simulink model "IEEE30_case"  (R2024b)
settings: Solver=FixedStepAuto  StartTime=0  StopTime=5  FixedStep=1e-7  RelTol=1e-3
values from neighbouring files (symbols this model uses):
  GFL_DFIG_7_C_bus = 0.08    [IEEE30_case_parameters.m]
  GFL_DFIG_7_D_mutual = 2.500000e+3    (= 2500)    [IEEE30_case_parameters.m]
  GFL_DFIG_7_f0 = 60    [IEEE30_case_parameters.m]
  GFL_DFIG_7_gPLLi = 3200    [IEEE30_case_parameters.m]
  GFL_DFIG_7_gPLLp = 650    [IEEE30_case_parameters.m]
  GFL_DFIG_7_H_WT = 0.4    [IEEE30_case_parameters.m]
  GFL_DFIG_7_Hg = 0.8    [IEEE30_case_parameters.m]
  GFL_DFIG_7_Igq_ref = 0    [IEEE30_case_parameters.m]
  GFL_DFIG_7_Ird_ref = 704.45696    [IEEE30_case_parameters.m]
  GFL_DFIG_7_KI_V = -300000    [IEEE30_case_parameters.m]
  GFL_DFIG_7_KP_V = -1000    [IEEE30_case_parameters.m]
  GFL_DFIG_7_Ksh = 1.254300e+4    (= 12543)    [IEEE30_case_parameters.m]
  GFL_DFIG_7_Lg = 0.000483    [IEEE30_case_parameters.m]
  GFL_DFIG_7_Lm_pu = 4    [IEEE30_case_parameters.m]
  GFL_DFIG_7_N = 100    [IEEE30_case_parameters.m]
  GFL_DFIG_7_p = 2    [IEEE30_case_parameters.m]
  GFL_DFIG_7_Pitch = 0    [IEEE30_case_parameters.m]
  GFL_DFIG_7_R = 44    [IEEE30_case_parameters.m]
  GFL_DFIG_7_Rg = 2.000000e-5    (= 2e-05)    [IEEE30_case_parameters.m]
  GFL_DFIG_7_rho = 1.225    [IEEE30_case_parameters.m]
  GFL_DFIG_7_rPLLi = 4500    [IEEE30_case_parameters.m]
  GFL_DFIG_7_rPLLp = 620    [IEEE30_case_parameters.m]
  GFL_DFIG_7_Rs_pu = 0.011    [IEEE30_case_parameters.m]
  GFL_DFIG_7_Sbase = 2.000000e+6    (= 2000000)    [IEEE30_case_parameters.m]
  GFL_DFIG_7_ugq_ref = 0    [IEEE30_case_parameters.m]
  GFL_DFIG_7_usd_ref = 0    [IEEE30_case_parameters.m]
  GFL_DFIG_7_Vbase = 690    [IEEE30_case_parameters.m]
  GFL_DFIG_7_Vdc_ref = 1200    [IEEE30_case_parameters.m]
  GFL_DFIG_7_wind = 12    [IEEE30_case_parameters.m]
  GFL_DFIG_7_wm_ref = 518.184209    [IEEE30_case_parameters.m]
  SG_D_13_D = 0.01056    [IEEE30_case_parameters.m]
  SG_D_13_EnableSaturation = 0    [IEEE30_case_parameters.m]
  SG_D_13_f0 = 60    [IEEE30_case_parameters.m]
  SG_D_13_H = 7.5    [IEEE30_case_parameters.m]
  SG_D_13_K_A = 20    [IEEE30_case_parameters.m]
  SG_D_13_K_E = 1.000000e+1    (= 10)    [IEEE30_case_parameters.m]
  SG_D_13_K_F = 2.363    [IEEE30_case_parameters.m]
  SG_D_13_K_s = 0.5    [IEEE30_case_parameters.m]
  SG_D_13_R_a = 0.001088    [IEEE30_case_parameters.m]
  SG_D_13_S_A = 1    [IEEE30_case_parameters.m]
  SG_D_13_S_B = 0.103    [IEEE30_case_parameters.m]
  SG_D_13_S_N = 10.659857    [IEEE30_case_parameters.m]
  SG_D_13_SpeedPara = 200    [IEEE30_case_parameters.m]
  SG_D_13_T_0 = 0.370163    [IEEE30_case_parameters.m]
  SG_D_13_T_1 = 0.3    [IEEE30_case_parameters.m]
  SG_D_13_T_2 = 0.05    [IEEE30_case_parameters.m]
  SG_D_13_T_3 = 0.02    [IEEE30_case_parameters.m]
  SG_D_13_T_4 = 0.005    [IEEE30_case_parameters.m]
  SG_D_13_T_A = 0.02    [IEEE30_case_parameters.m]
  SG_D_13_T_dd = 8.000000e+0    (= 8)    [IEEE30_case_parameters.m]
  SG_D_13_T_ddd = 0.04    [IEEE30_case_parameters.m]
  SG_D_13_T_E = 0.314    [IEEE30_case_parameters.m]
  SG_D_13_T_F = 0.35    [IEEE30_case_parameters.m]
  SG_D_13_T_qd = 0.8    [IEEE30_case_parameters.m]
  SG_D_13_T_qdd = 0.02    [IEEE30_case_parameters.m]
  SG_D_13_T_speed = 0.1    [IEEE30_case_parameters.m]
  SG_D_13_T_w = 0.5    [IEEE30_case_parameters.m]
  SG_D_13_V_ref = 1.696619    [IEEE30_case_parameters.m]
  SG_D_13_w_ref = 376.991118    [IEEE30_case_parameters.m]
  SG_D_13_x_d = 1.9    [IEEE30_case_parameters.m]
  SG_D_13_x_dd = 0.302    [IEEE30_case_parameters.m]
  SG_D_13_x_ddd = 0.204    [IEEE30_case_parameters.m]
  SG_D_13_x_l = 0.05    [IEEE30_case_parameters.m]
  SG_D_13_x_q = 1.3    [IEEE30_case_parameters.m]
  SG_D_13_x_qd = 0.5    [IEEE30_case_parameters.m]
  SG_D_13_x_qdd = 0.3    [IEEE30_case_parameters.m]
  SG_D_1_D = 0.01056    [IEEE30_case_parameters.m]
  SG_D_1_EnableSaturation = 0    [IEEE30_case_parameters.m]
  SG_D_1_f0 = 60    [IEEE30_case_parameters.m]
  SG_D_1_H = 7.5    [IEEE30_case_parameters.m]
  SG_D_1_K_A = 20    [IEEE30_case_parameters.m]
  SG_D_1_K_E = 1.000000e+1    (= 10)    [IEEE30_case_parameters.m]
  SG_D_1_K_F = 2.363    [IEEE30_case_parameters.m]
  SG_D_1_K_s = 0.5    [IEEE30_case_parameters.m]
  SG_D_1_R_a = 0.001088    [IEEE30_case_parameters.m]
  SG_D_1_S_A = 1    [IEEE30_case_parameters.m]
  SG_D_1_S_B = 0.103    [IEEE30_case_parameters.m]
  SG_D_1_S_N = 10.659857    [IEEE30_case_parameters.m]
  SG_D_1_SpeedPara = 200    [IEEE30_case_parameters.m]
  SG_D_1_T_0 = 0.259812    [IEEE30_case_parameters.m]
  SG_D_1_T_1 = 0.3    [IEEE30_case_parameters.m]
  SG_D_1_T_2 = 0.05    [IEEE30_case_parameters.m]
  SG_D_1_T_3 = 0.02    [IEEE30_case_parameters.m]
  SG_D_1_T_4 = 0.005    [IEEE30_case_parameters.m]
  SG_D_1_T_A = 0.02    [IEEE30_case_parameters.m]
  SG_D_1_T_dd = 8.000000e+0    (= 8)    [IEEE30_case_parameters.m]
  SG_D_1_T_ddd = 0.04    [IEEE30_case_parameters.m]
  SG_D_1_T_E = 0.314    [IEEE30_case_parameters.m]
  SG_D_1_T_F = 0.35    [IEEE30_case_parameters.m]
  SG_D_1_T_qd = 0.8    [IEEE30_case_parameters.m]
  SG_D_1_T_qdd = 0.02    [IEEE30_case_parameters.m]
  SG_D_1_T_speed = 0.1    [IEEE30_case_parameters.m]
  SG_D_1_T_w = 0.5    [IEEE30_case_parameters.m]
  SG_D_1_V_ref = 1.544107    [IEEE30_case_parameters.m]
  SG_D_1_w_ref = 376.991118    [IEEE30_case_parameters.m]
  SG_D_1_x_d = 1.9    [IEEE30_case_parameters.m]
  SG_D_1_x_dd = 0.302    [IEEE30_case_parameters.m]
  SG_D_1_x_ddd = 0.204    [IEEE30_case_parameters.m]
  SG_D_1_x_l = 0.05    [IEEE30_case_parameters.m]
  SG_D_1_x_q = 1.3    [IEEE30_case_parameters.m]
  SG_D_1_x_qd = 0.5    [IEEE30_case_parameters.m]
  SG_D_1_x_qdd = 0.3    [IEEE30_case_parameters.m]
  SG_D_22_D = 0.01056    [IEEE30_case_parameters.m]
  SG_D_22_EnableSaturation = 0    [IEEE30_case_parameters.m]
  SG_D_22_f0 = 60    [IEEE30_case_parameters.m]
  SG_D_22_H = 7.5    [IEEE30_case_parameters.m]
  SG_D_22_K_A = 20    [IEEE30_case_parameters.m]
  SG_D_22_K_E = 1.000000e+1    (= 10)    [IEEE30_case_parameters.m]
  SG_D_22_K_F = 2.363    [IEEE30_case_parameters.m]
  SG_D_22_K_s = 0.5    [IEEE30_case_parameters.m]
  SG_D_22_R_a = 0.001088    [IEEE30_case_parameters.m]
  SG_D_22_S_A = 1    [IEEE30_case_parameters.m]
  SG_D_22_S_B = 0.103    [IEEE30_case_parameters.m]
  SG_D_22_S_N = 10.659857    [IEEE30_case_parameters.m]
  SG_D_22_SpeedPara = 200    [IEEE30_case_parameters.m]
  SG_D_22_T_0 = 0.216121    [IEEE30_case_parameters.m]
  SG_D_22_T_1 = 0.3    [IEEE30_case_parameters.m]
  SG_D_22_T_2 = 0.05    [IEEE30_case_parameters.m]
  SG_D_22_T_3 = 0.02    [IEEE30_case_parameters.m]
  SG_D_22_T_4 = 0.005    [IEEE30_case_parameters.m]
  ... (+126 more)
(part 21 of 27)

== system IEEE30_case/SG_D_2/d_w_SG_D_2_block ==
  note: d_w_SG_D_2 in IEEE30_case
      | $\frac{2\,\pi \,T_{m,\mathrm{SG},D,2}\,f_{0}-D\,\left(w_{\mathrm{SG},D,2}-2\,\pi \,f_{0}\right)+2\,\pi \,f_{0}\,\left(\frac{\psi _{d,\mathrm{SG},D,2}\,\left(\psi _{q,\mathrm{SG},D,2}+\frac{\psi _{\mathrm{gq},\mathrm{SG},D,2}\,\left(x_{l}-x_{\mathrm{qdd}}\right)}{x_{l}-x_{\mathrm{qd}}}+\frac{\psi _{\mathrm{kq},\mathrm{SG},D,2}\,\left(x_{\mathrm{qd}}-x_{\mathrm{qdd}}\right)}{x_{l}-x_{\mathrm{qd}}}\right)}{x_{\mathrm{qdd}}}+\frac{\psi _{q,\mathrm{SG},D,2}\,\left(\frac{\psi _{\mathrm{1d},\mathrm{SG},D,2}\,\left(x_{\mathrm{dd}}-x_{\mathrm{ddd}}\right)}{x_{\mathrm{dd}}-x_{l}}-\psi _{d,\mathrm{SG},D,2}+\frac{\psi _{\mathrm{fd},\mathrm{SG},D,2}\,\left(x_{\mathrm{ddd}}-x_{l}\right)}{x_{\mathrm{dd}}-x_{l}}\right)}{x_{\mathrm{ddd}}}\right)}{2\,H}$
      | Automatically generated on 2025-11-01 18:31:31 .
  State_w_SG_D_2_071c4 : Inport
  State_T_m_SG_D_2_860e5 : Inport  Port=2
  State_psi_d_SG_D_2_34ede : Inport  Port=3
  State_psi_gq_SG_D_2_9f73e : Inport  Port=4
  State_psi_kq_SG_D_2_c590e : Inport  Port=5
  State_psi_q_SG_D_2_76d6b : Inport  Port=6
  State_psi_q_SG_D_2_b0e4a : Inport  Port=7
  State_psi_1d_SG_D_2_97ed5 : Inport  Port=8
  State_psi_d_SG_D_2_9b8cf : Inport  Port=9
  State_psi_fd_SG_D_2_66d61 : Inport  Port=10
  Add_2de3b : Sum
  Add_3480c : Sum
  Add_48811 : Sum
  Add_490e2 : Sum
  Add_ac965 : Sum
  Add_c5c05 : Sum
  Add_cbfef : Sum
  Add_e3b53 : Sum
  Constant_-1_0f227 : Constant  Value=-1
  Constant_-1_31bfd : Constant  Value=-1
  Constant_-1_403be : Constant  Value=-1
  Constant_-1_8cfa0 : Constant  Value=-1
  Constant_-1_aa771 : Constant  Value=-1
  Constant_-1_c9d01 : Constant  Value=-1
  Constant_-2.0_e1ab0 : Constant  Value=-2.0
  Constant_2.0_7b2d5 : Constant  Value=2.0
  Constant_2.0_88953 : Constant  Value=2.0
  Constant_2.0_a1518 : Constant  Value=2.0
  Constant_D_aefe5 : Constant  Value=D
  Constant_H_d5073 : Constant  Value=H
  Constant_f0_92636 : Constant  Value=f0
  Constant_f0_969d1 : Constant  Value=f0
  Constant_f0_ac18e : Constant  Value=f0
  Constant_pi_a4aaa : Constant  Value=pi
  Constant_pi_ba27e : Constant  Value=pi
  Constant_pi_e4e5a : Constant  Value=pi
  Constant_x_dd_04dea : Constant  Value=x_dd
  Constant_x_dd_1dd6c : Constant  Value=x_dd
  Constant_x_dd_c91bf : Constant  Value=x_dd
  Constant_x_ddd_2aedd : Constant  Value=x_ddd
  Constant_x_ddd_ab5ce : Constant  Value=x_ddd
  Constant_x_ddd_af871 : Constant  Value=x_ddd
  Constant_x_l_51bc5 : Constant  Value=x_l
  Constant_x_l_9b514 : Constant  Value=x_l
  Constant_x_l_9de80 : Constant  Value=x_l
  Constant_x_l_b1654 : Constant  Value=x_l
  Constant_x_l_d50ef : Constant  Value=x_l
  Constant_x_l_e71a3 : Constant  Value=x_l
  Constant_x_qd_83da6 : Constant  Value=x_qd
  Constant_x_qd_c91d9 : Constant  Value=x_qd
  Constant_x_qd_f6865 : Constant  Value=x_qd
  Constant_x_qdd_13a68 : Constant  Value=x_qdd
  Constant_x_qdd_65572 : Constant  Value=x_qdd
  Constant_x_qdd_d4bb8 : Constant  Value=x_qdd
  Divide_24348 : Product  Inputs=*/
  Divide_4956c : Product  Inputs=*/
  Divide_b34f4 : Product  Inputs=*/
  Divide_c5fd0 : Product  Inputs=*/
  Divide_df850 : Product  Inputs=*/
  Divide_edb71 : Product  Inputs=*/
  Divide_f021f : Product  Inputs=*/
  Product_08d4b : Product
  Product_17292 : Product
  Product_197e6 : Product
  Product_46ca4 : Product
  Product_50005 : Product
  Product_567dd : Product
  Product_57114 : Product
  Product_67bf0 : Product
  Product_775d5 : Product
  Product_7a3b7 : Product
  Product_9210e : Product
  Product_934a5 : Product
  Product_b04a5 : Product
  Product_b6084 : Product
  Product_b7d0d : Product
  Product_cd995 : Product
  Product_d2ecf : Product
  Product_deb05 : Product
  Product_e6081 : Product
  Product_e630b : Product
  Product_eaea2 : Product
  Product_ed81a : Product
  Subtract_0b144 : Sum  Inputs=+-
  Subtract_0e36e : Sum  Inputs=+-
  Subtract_4b2ef : Sum  Inputs=+-
  Subtract_59a92 : Sum  Inputs=+-
  Subtract_5b0ec : Sum  Inputs=+-
  Subtract_8ba6d : Sum  Inputs=+-
  Subtract_9d6d9 : Sum  Inputs=+-
  Subtract_b5e26 : Sum  Inputs=+-
  Blockout_d_w_SG_D_2_6b1c2 : Outport
  wires:
  Constant_x_qd_c91d9/1 -> Subtract_9d6d9/1
  Constant_-1_c9d01/1 -> Product_cd995/1
  Constant_-1_403be/1 -> Product_e630b/1
  Constant_x_qdd_65572/1 -> Subtract_9d6d9/2
  Subtract_b5e26/1 -> Divide_b34f4/2
  Constant_x_l_9b514/1 -> Product_cd995/2
  Constant_x_l_e71a3/1 -> Product_e630b/2
  Product_cd995/1 -> Add_ac965/1
  Product_e630b/1 -> Add_2de3b/1
  Constant_x_l_9de80/1 -> Subtract_4b2ef/2
  Constant_x_l_b1654/1 -> Product_b6084/2
  Constant_x_ddd_af871/1 -> Divide_24348/2
  Subtract_5b0ec/1 -> Product_934a5/2
  Constant_x_qd_f6865/1 -> Add_ac965/2
  Constant_x_qdd_d4bb8/1 -> Add_2de3b/2
  Constant_-1_aa771/1 -> Product_b6084/1
  State_psi_d_SG_D_2_34ede/1 -> Product_50005/2
  Constant_-1_8cfa0/1 -> Product_67bf0/1
  State_w_SG_D_2_071c4/1 -> Add_c5c05/2
  Product_b6084/1 -> Add_e3b53/1
  State_psi_1d_SG_D_2_97ed5/1 -> Product_67bf0/2
  Constant_x_dd_04dea/1 -> Subtract_59a92/1
  Divide_c5fd0/1 -> Subtract_0e36e/1
  Subtract_9d6d9/1 -> Product_567dd/2
  Constant_x_ddd_2aedd/1 -> Subtract_59a92/2
  State_psi_gq_SG_D_2_9f73e/1 -> Product_ed81a/1
  Add_ac965/1 -> Divide_edb71/2
  State_psi_d_SG_D_2_9b8cf/1 -> Add_cbfef/2
  Add_2de3b/1 -> Product_ed81a/2
  Constant_x_qd_83da6/1 -> Add_e3b53/2
  State_psi_kq_SG_D_2_c590e/1 -> Product_567dd/1
  Product_67bf0/1 -> Product_17292/1
  Subtract_59a92/1 -> Product_17292/2
  Constant_pi_a4aaa/1 -> Product_d2ecf/2
  Constant_x_dd_1dd6c/1 -> Subtract_4b2ef/1
  Constant_x_ddd_ab5ce/1 -> Subtract_5b0ec/1
  Constant_x_l_d50ef/1 -> Subtract_5b0ec/2
  Product_ed81a/1 -> Divide_c5fd0/1
  Add_e3b53/1 -> Divide_c5fd0/2
  Add_490e2/1 -> Product_197e6/2
  Product_567dd/1 -> Divide_edb71/1
  Constant_pi_e4e5a/1 -> Product_46ca4/2
  Product_17292/1 -> Divide_f021f/1
  Subtract_4b2ef/1 -> Divide_f021f/2
  State_psi_fd_SG_D_2_66d61/1 -> Product_934a5/1
  Divide_f021f/1 -> Add_cbfef/1
  Constant_x_dd_c91bf/1 -> Subtract_b5e26/1
  Constant_x_l_51bc5/1 -> Subtract_b5e26/2
  Divide_edb71/1 -> Subtract_0e36e/2
  Product_934a5/1 -> Divide_b34f4/1
  Constant_-1_0f227/1 -> Product_50005/1
  Constant_-2.0_e1ab0/1 -> Product_46ca4/1
  Subtract_0e36e/1 -> Add_490e2/1
  Subtract_8ba6d/1 -> Product_b7d0d/2
  State_psi_q_SG_D_2_76d6b/1 -> Add_490e2/2
  Constant_D_aefe5/1 -> Product_e6081/2
  Add_cbfef/1 -> Subtract_8ba6d/1
  Divide_b34f4/1 -> Subtract_8ba6d/2
  Product_46ca4/1 -> Product_775d5/1
  Constant_f0_92636/1 -> Product_775d5/2
  Constant_2.0_88953/1 -> Product_d2ecf/1
  Product_50005/1 -> Product_197e6/1
  State_psi_q_SG_D_2_b0e4a/1 -> Product_b7d0d/1
  Constant_-1_31bfd/1 -> Product_e6081/1
  Product_775d5/1 -> Add_c5c05/1
  Product_d2ecf/1 -> Product_08d4b/1
  State_T_m_SG_D_2_860e5/1 -> Product_08d4b/2
  Constant_2.0_a1518/1 -> Product_9210e/1
  Constant_pi_ba27e/1 -> Product_9210e/2
  Product_197e6/1 -> Divide_df850/1
  Constant_x_qdd_13a68/1 -> Divide_df850/2
  Product_b7d0d/1 -> Divide_24348/1
  Product_e6081/1 -> Product_eaea2/1
  Add_c5c05/1 -> Product_eaea2/2
  Product_08d4b/1 -> Product_57114/1
  Constant_f0_ac18e/1 -> Product_57114/2
  Product_9210e/1 -> Product_deb05/1
  Constant_f0_969d1/1 -> Product_deb05/2
  Divide_df850/1 -> Add_3480c/1
  Divide_24348/1 -> Add_3480c/2
  Product_eaea2/1 -> Add_48811/1
  Product_57114/1 -> Add_48811/2
  Product_deb05/1 -> Product_7a3b7/1
  Add_3480c/1 -> Product_7a3b7/2
  Add_48811/1 -> Subtract_0b144/1
  Product_7a3b7/1 -> Subtract_0b144/2
  Constant_2.0_7b2d5/1 -> Product_b04a5/1
  Constant_H_d5073/1 -> Product_b04a5/2
  Subtract_0b144/1 -> Divide_4956c/1
  Product_b04a5/1 -> Divide_4956c/2
  Divide_4956c/1 -> Blockout_d_w_SG_D_2_6b1c2/1

== system IEEE30_case/SG_D_2/i_d_SG_D_2_block ==
  note: i_d_SG_D_2 in IEEE30_case
      | $\frac{\sin\left(\theta _{\mathrm{SG},D,2}\right)\,\left(\frac{\psi _{\mathrm{1d},\mathrm{SG},D,2}\,\left(x_{\mathrm{dd}}-x_{\mathrm{ddd}}\right)}{x_{\mathrm{dd}}-x_{l}}-\psi _{d,\mathrm{SG},D,2}+\frac{\psi _{\mathrm{fd},\mathrm{SG},D,2}\,\left(x_{\mathrm{ddd}}-x_{l}\right)}{x_{\mathrm{dd}}-x_{l}}\right)}{x_{\mathrm{ddd}}}-\frac{\cos\left(\theta _{\mathrm{SG},D,2}\right)\,\left(\psi _{q,\mathrm{SG},D,2}+\frac{\psi _{\mathrm{gq},\mathrm{SG},D,2}\,\left(x_{l}-x_{\mathrm{qdd}}\right)}{x_{l}-x_{\mathrm{qd}}}+\frac{\psi _{\mathrm{kq},\mathrm{SG},D,2}\,\left(x_{\mathrm{qd}}-x_{\mathrm{qdd}}\right)}{x_{l}-x_{\mathrm{qd}}}\right)}{x_{\mathrm{qdd}}}$
      | Automatically generated on 2025-11-01 18:31:53 .
  State_psi_gq_SG_D_2_ef87c : Inport
  State_psi_kq_SG_D_2_da414 : Inport  Port=2
  State_psi_q_SG_D_2_14a65 : Inport  Port=3
  State_theta_SG_D_2_b0b05 : Inport  Port=4
  State_psi_1d_SG_D_2_baa39 : Inport  Port=5
  State_psi_d_SG_D_2_956af : Inport  Port=6
  State_psi_fd_SG_D_2_52aed : Inport  Port=7
  State_theta_SG_D_2_57fa8 : Inport  Port=8
  Add_190e7 : Sum
  Add_2cec0 : Sum
  Add_5ba1c : Sum
  Add_e5908 : Sum
  Add_f3d0a : Sum
  Constant_-1_2e41f : Constant  Value=-1
  Constant_-1_404a3 : Constant  Value=-1
  Constant_-1_80a87 : Constant  Value=-1
  Constant_-1_f25b1 : Constant  Value=-1
  Constant_-1_f5693 : Constant  Value=-1
  Constant_x_dd_2d4e9 : Constant  Value=x_dd
  Constant_x_dd_42557 : Constant  Value=x_dd
  Constant_x_dd_b8c41 : Constant  Value=x_dd
  Constant_x_ddd_2c46a : Constant  Value=x_ddd
  Constant_x_ddd_8aad1 : Constant  Value=x_ddd
  Constant_x_ddd_95243 : Constant  Value=x_ddd
  Constant_x_l_08223 : Constant  Value=x_l
  Constant_x_l_355f8 : Constant  Value=x_l
  Constant_x_l_559b2 : Constant  Value=x_l
  Constant_x_l_b22e8 : Constant  Value=x_l
  Constant_x_l_d52ee : Constant  Value=x_l
  Constant_x_l_e61e2 : Constant  Value=x_l
  Constant_x_qd_3c262 : Constant  Value=x_qd
  Constant_x_qd_5b82d : Constant  Value=x_qd
  Constant_x_qd_da69c : Constant  Value=x_qd
  Constant_x_qdd_1f1d5 : Constant  Value=x_qdd
  Constant_x_qdd_3610f : Constant  Value=x_qdd
  Constant_x_qdd_cad96 : Constant  Value=x_qdd
  Divide_32941 : Product  Inputs=*/
  Divide_3dcdd : Product  Inputs=*/
  Divide_9da8b : Product  Inputs=*/
  Divide_aeac0 : Product  Inputs=*/
  Divide_c0da5 : Product  Inputs=*/
  Divide_e74a2 : Product  Inputs=*/
  MathFunc_cos_8df34 : Trigonometry  Operator=cos
  MathFunc_sin_f790c : Trigonometry
  Product_11a30 : Product
  Product_11e29 : Product
  Product_2653c : Product
  Product_2b1e0 : Product
  Product_3265d : Product
  Product_3d1f3 : Product
  Product_4bdee : Product
  Product_60792 : Product
  Product_af2fe : Product
  Product_ba15b : Product
  Product_d1e53 : Product
  Subtract_38201 : Sum  Inputs=+-
  Subtract_4005b : Sum  Inputs=+-
  Subtract_7917b : Sum  Inputs=+-
  Subtract_90c1d : Sum  Inputs=+-
  Subtract_9241a : Sum  Inputs=+-
  Subtract_92dc1 : Sum  Inputs=+-
  Subtract_b4de5 : Sum  Inputs=+-
  Subtract_e026e : Sum  Inputs=+-
  Blockout_i_d_SG_D_2_ae2df : Outport
  wires:
  Constant_x_ddd_2c46a/1 -> Subtract_b4de5/1
  Constant_x_qd_da69c/1 -> Subtract_38201/1
  Constant_-1_80a87/1 -> Product_af2fe/1
  Constant_-1_f25b1/1 -> Product_3d1f3/1
  Subtract_9241a/1 -> Blockout_i_d_SG_D_2_ae2df/1
  Constant_x_qdd_cad96/1 -> Subtract_38201/2
  Constant_x_l_b22e8/1 -> Product_af2fe/2
  Constant_x_l_559b2/1 -> Product_3d1f3/2
  Product_af2fe/1 -> Add_f3d0a/1
  Product_3d1f3/1 -> Add_2cec0/1
  Constant_x_l_355f8/1 -> Product_2b1e0/2
  Constant_x_qd_5b82d/1 -> Add_f3d0a/2
  Constant_x_qdd_3610f/1 -> Add_2cec0/2
  Constant_x_qdd_1f1d5/1 -> Divide_c0da5/2
  MathFunc_cos_8df34/1 -> Product_3265d/2
  Constant_-1_404a3/1 -> Product_2b1e0/1
  State_psi_gq_SG_D_2_ef87c/1 -> Product_4bdee/1
  Subtract_b4de5/1 -> Product_11e29/2
  Product_ba15b/1 -> Product_2653c/1
  Add_f3d0a/1 -> Divide_9da8b/2
  Add_2cec0/1 -> Product_4bdee/2
  Product_11e29/1 -> Divide_3dcdd/1
  Product_2b1e0/1 -> Add_5ba1c/1
  Constant_x_qd_3c262/1 -> Add_5ba1c/2
  State_theta_SG_D_2_57fa8/1 -> MathFunc_sin_f790c/1
  State_psi_kq_SG_D_2_da414/1 -> Product_60792/1
  Add_190e7/1 -> Subtract_92dc1/1
  Subtract_38201/1 -> Product_60792/2
  Product_4bdee/1 -> Divide_e74a2/1
  Constant_-1_f5693/1 -> Product_ba15b/1
  State_psi_1d_SG_D_2_baa39/1 -> Product_ba15b/2
  State_psi_fd_SG_D_2_52aed/1 -> Product_11e29/1
  Constant_x_dd_b8c41/1 -> Subtract_e026e/1
  Product_2653c/1 -> Divide_aeac0/1
  Constant_x_ddd_95243/1 -> Subtract_e026e/2
  Divide_3dcdd/1 -> Subtract_92dc1/2
  Add_5ba1c/1 -> Divide_e74a2/2
  Product_11a30/1 -> Divide_32941/1
  Product_60792/1 -> Divide_9da8b/1
  Constant_-1_2e41f/1 -> Product_d1e53/1
  Subtract_4005b/1 -> Divide_3dcdd/2
  Subtract_e026e/1 -> Product_2653c/2
  Constant_x_dd_2d4e9/1 -> Subtract_7917b/1
  Subtract_92dc1/1 -> Product_11a30/1
  Constant_x_l_d52ee/1 -> Subtract_7917b/2
  Constant_x_l_08223/1 -> Subtract_b4de5/2
  Divide_e74a2/1 -> Subtract_90c1d/1
  Divide_32941/1 -> Subtract_9241a/2
  Divide_9da8b/1 -> Subtract_90c1d/2
  Subtract_7917b/1 -> Divide_aeac0/2
  Constant_x_dd_42557/1 -> Subtract_4005b/1
  Divide_c0da5/1 -> Subtract_9241a/1
  Constant_x_l_e61e2/1 -> Subtract_4005b/2
  Subtract_90c1d/1 -> Add_e5908/1
  State_psi_q_SG_D_2_14a65/1 -> Add_e5908/2
  Constant_x_ddd_8aad1/1 -> Divide_32941/2
  MathFunc_sin_f790c/1 -> Product_11a30/2
  Divide_aeac0/1 -> Add_190e7/1
  State_psi_d_SG_D_2_956af/1 -> Add_190e7/2
  Add_e5908/1 -> Product_d1e53/2
  State_theta_SG_D_2_b0b05/1 -> MathFunc_cos_8df34/1
  Product_d1e53/1 -> Product_3265d/1
  Product_3265d/1 -> Divide_c0da5/1

== system IEEE30_case/SG_D_2/i_q_SG_D_2_block ==
  note: i_q_SG_D_2 in IEEE30_case
      | $-\frac{\sin\left(\theta _{\mathrm{SG},D,2}\right)\,\left(\psi _{q,\mathrm{SG},D,2}+\frac{\psi _{\mathrm{gq},\mathrm{SG},D,2}\,\left(x_{l}-x_{\mathrm{qdd}}\right)}{x_{l}-x_{\mathrm{qd}}}+\frac{\psi _{\mathrm{kq},\mathrm{SG},D,2}\,\left(x_{\mathrm{qd}}-x_{\mathrm{qdd}}\right)}{x_{l}-x_{\mathrm{qd}}}\right)}{x_{\mathrm{qdd}}}-\frac{\cos\left(\theta _{\mathrm{SG},D,2}\right)\,\left(\frac{\psi _{\mathrm{1d},\mathrm{SG},D,2}\,\left(x_{\mathrm{dd}}-x_{\mathrm{ddd}}\right)}{x_{\mathrm{dd}}-x_{l}}-\psi _{d,\mathrm{SG},D,2}+\frac{\psi _{\mathrm{fd},\mathrm{SG},D,2}\,\left(x_{\mathrm{ddd}}-x_{l}\right)}{x_{\mathrm{dd}}-x_{l}}\right)}{x_{\mathrm{ddd}}}$
      | Automatically generated on 2025-11-01 18:31:57 .
  State_psi_gq_SG_D_2_0f140 : Inport
  State_psi_kq_SG_D_2_8caff : Inport  Port=2
  State_psi_q_SG_D_2_c9d02 : Inport  Port=3
  State_theta_SG_D_2_99776 : Inport  Port=4
  State_psi_1d_SG_D_2_3670e : Inport  Port=5
  State_psi_d_SG_D_2_82684 : Inport  Port=6
  State_psi_fd_SG_D_2_4cfda : Inport  Port=7
  State_theta_SG_D_2_e3ac6 : Inport  Port=8
  Add_18b6d : Sum
  Add_1d44b : Sum
  Add_3a2b5 : Sum
  Add_9698d : Sum
  Add_9d5bd : Sum
  Add_e2752 : Sum
  Constant_-1_{46827,56218,94343,94462} (4 alike) : Constant  Value=-1
  Constant_-1_50b0c : Constant  Value=-1
  Constant_x_dd_09e07 : Constant  Value=x_dd
  Constant_x_dd_77471 : Constant  Value=x_dd
  Constant_x_dd_79e24 : Constant  Value=x_dd
  Constant_x_ddd_2d654 : Constant  Value=x_ddd
  Constant_x_ddd_4337c : Constant  Value=x_ddd
  Constant_x_ddd_5f735 : Constant  Value=x_ddd
  Constant_x_l_433ef : Constant  Value=x_l
  Constant_x_l_4ca2f : Constant  Value=x_l
  Constant_x_l_5195e : Constant  Value=x_l
  Constant_x_l_a3f6e : Constant  Value=x_l
  Constant_x_l_ab249 : Constant  Value=x_l
  Constant_x_l_b7b4e : Constant  Value=x_l
  Constant_x_qd_4d715 : Constant  Value=x_qd
  Constant_x_qd_58a0f : Constant  Value=x_qd
  Constant_x_qd_6d9e4 : Constant  Value=x_qd
  Constant_x_qdd_3f9be : Constant  Value=x_qdd
  Constant_x_qdd_ae7a5 : Constant  Value=x_qdd
  Constant_x_qdd_ebd74 : Constant  Value=x_qdd
  Divide_05f23 : Product  Inputs=*/
  Divide_2a0fd : Product  Inputs=*/
  Divide_4fdbe : Product  Inputs=*/
  Divide_6d0b3 : Product  Inputs=*/
  Divide_b374c : Product  Inputs=*/
  Divide_f150f : Product  Inputs=*/
  MathFunc_cos_a52ff : Trigonometry  Operator=cos
  MathFunc_sin_0fb9d : Trigonometry
  Product_02529 : Product
  Product_03870 : Product
  Product_2e37c : Product
  Product_4d747 : Product
  Product_4d981 : Product
  Product_59f12 : Product
  Product_a5dfa : Product
  Product_ad008 : Product
  Product_b383d : Product
  Product_f4942 : Product
  Product_f5289 : Product
  Subtract_01e2a : Sum  Inputs=+-
  Subtract_1994f : Sum  Inputs=+-
  Subtract_608a5 : Sum  Inputs=+-
  Subtract_78221 : Sum  Inputs=+-
  Subtract_a0408 : Sum  Inputs=+-
  Subtract_abee3 : Sum  Inputs=+-
  Subtract_e9404 : Sum  Inputs=+-
  Blockout_i_q_SG_D_2_865bf : Outport
  wires:
  MathFunc_sin_0fb9d/1 -> Product_f4942/2
  Product_b383d/1 -> Product_f4942/1
  Constant_-1_56218/1 -> Product_ad008/1
  Constant_-1_94462/1 -> Product_2e37c/1
  Constant_x_l_a3f6e/1 -> Product_ad008/2
  Product_ad008/1 -> Add_9d5bd/1
  Subtract_78221/1 -> Product_03870/2
  Constant_x_qdd_ebd74/1 -> Subtract_1994f/2
  Constant_x_qdd_3f9be/1 -> Add_9d5bd/2
  Add_3a2b5/1 -> Product_b383d/2
  Constant_x_l_4ca2f/1 -> Product_2e37c/2
  Constant_x_qd_6d9e4/1 -> Subtract_1994f/1
  Constant_-1_46827/1 -> Product_59f12/1
  Constant_x_l_433ef/1 -> Product_59f12/2
  State_psi_1d_SG_D_2_3670e/1 -> Product_a5dfa/2
  State_psi_gq_SG_D_2_0f140/1 -> Product_02529/1
  Add_9d5bd/1 -> Product_02529/2
  Product_2e37c/1 -> Add_1d44b/1
  Divide_05f23/1 -> Add_18b6d/1
  Constant_x_qd_58a0f/1 -> Add_1d44b/2
  State_psi_kq_SG_D_2_8caff/1 -> Product_f5289/1
  Add_9698d/1 -> Subtract_abee3/1
  Constant_x_ddd_4337c/1 -> Subtract_78221/2
  Subtract_1994f/1 -> Product_f5289/2
  Product_59f12/1 -> Add_e2752/1
  Constant_x_qd_4d715/1 -> Add_e2752/2
  Constant_-1_94343/1 -> Product_a5dfa/1
  Constant_x_l_b7b4e/1 -> Subtract_e9404/2
  Constant_x_dd_79e24/1 -> Subtract_78221/1
  Product_02529/1 -> Divide_6d0b3/1
  Divide_4fdbe/1 -> Subtract_abee3/2
  Add_1d44b/1 -> Divide_6d0b3/2
  Product_4d981/1 -> Divide_b374c/1
  Product_f5289/1 -> Divide_f150f/1
  Constant_-1_50b0c/1 -> Product_b383d/1
  Product_a5dfa/1 -> Product_03870/1
  Add_e2752/1 -> Divide_f150f/2
  Constant_x_dd_77471/1 -> Subtract_608a5/1
  Subtract_abee3/1 -> Product_4d981/1
  Subtract_01e2a/1 -> Product_4d747/2
  Constant_x_l_5195e/1 -> Subtract_608a5/2
  Constant_x_ddd_5f735/1 -> Subtract_01e2a/1
  Constant_x_l_ab249/1 -> Subtract_01e2a/2
  Divide_6d0b3/1 -> Subtract_a0408/1
  Divide_b374c/1 -> Add_18b6d/2
  Product_4d747/1 -> Divide_4fdbe/1
  Divide_f150f/1 -> Subtract_a0408/2
  Subtract_e9404/1 -> Divide_4fdbe/2
  Product_03870/1 -> Divide_2a0fd/1
  Subtract_608a5/1 -> Divide_2a0fd/2
  Constant_x_qdd_ae7a5/1 -> Divide_05f23/2
  State_psi_fd_SG_D_2_4cfda/1 -> Product_4d747/1
  Constant_x_dd_09e07/1 -> Subtract_e9404/1
  Subtract_a0408/1 -> Add_3a2b5/1
  State_psi_q_SG_D_2_c9d02/1 -> Add_3a2b5/2
  Constant_x_ddd_2d654/1 -> Divide_b374c/2
  Divide_2a0fd/1 -> Add_9698d/1
  State_psi_d_SG_D_2_82684/1 -> Add_9698d/2
  State_theta_SG_D_2_99776/1 -> MathFunc_sin_0fb9d/1
  State_theta_SG_D_2_e3ac6/1 -> MathFunc_cos_a52ff/1
  MathFunc_cos_a52ff/1 -> Product_4d981/2
  Product_f4942/1 -> Divide_05f23/1
  Add_18b6d/1 -> Blockout_i_q_SG_D_2_865bf/1

== system IEEE30_case/SG_D_2/theta_SG_D_2_out_block ==
  note: theta_SG_D_2_out in IEEE30_case
      | $\theta _{\mathrm{SG},D,2}$
      | Automatically generated on 2025-11-01 18:32:02 .
  State_theta_SG_D_2_1ecf4 : Inport
  Blockout_theta_SG_D_2_out_e958d : Outport
  wires:
  State_theta_SG_D_2_1ecf4/1 -> Blockout_theta_SG_D_2_out_e958d/1

== system IEEE30_case/SG_D_2/w_SG_D_2_out_block ==
  note: w_SG_D_2_out in IEEE30_case
      | $w_{\mathrm{SG},D,2}$
      | Automatically generated on 2025-11-01 18:32:02 .
  State_w_SG_D_2_6b0c6 : Inport
  Blockout_w_SG_D_2_out_ca3f3 : Outport
  wires:
  State_w_SG_D_2_6b0c6/1 -> Blockout_w_SG_D_2_out_ca3f3/1

== system IEEE30_case/SG_D_22/T_e_SG_D_22_block ==
  note: T_e_SG_D_22 in IEEE30_case
      | $-\frac{\psi _{d,\mathrm{SG},D,22}\,\left(\psi _{q,\mathrm{SG},D,22}+\frac{\psi _{\mathrm{gq},\mathrm{SG},D,22}\,\left(x_{l}-x_{\mathrm{qdd}}\right)}{x_{l}-x_{\mathrm{qd}}}+\frac{\psi _{\mathrm{kq},\mathrm{SG},D,22}\,\left(x_{\mathrm{qd}}-x_{\mathrm{qdd}}\right)}{x_{l}-x_{\mathrm{qd}}}\right)}{x_{\mathrm{qdd}}}-\frac{\psi _{q,\mathrm{SG},D,22}\,\left(\frac{\psi _{\mathrm{1d},\mathrm{SG},D,22}\,\left(x_{\mathrm{dd}}-x_{\mathrm{ddd}}\right)}{x_{\mathrm{dd}}-x_{l}}-\psi _{d,\mathrm{SG},D,22}+\frac{\psi _{\mathrm{fd},\mathrm{SG},D,22}\,\left(x_{\mathrm{ddd}}-x_{l}\right)}{x_{\mathrm{dd}}-x_{l}}\right)}{x_{\mathrm{ddd}}}$
      | Automatically generated on 2025-11-01 18:36:46 .
  State_psi_d_SG_D_22_b0899 : Inport
  State_psi_gq_SG_D_22_ecb3d : Inport  Port=2
  State_psi_kq_SG_D_22_80cd8 : Inport  Port=3
  State_psi_q_SG_D_22_f98a6 : Inport  Port=4
  State_psi_q_SG_D_22_21d92 : Inport  Port=5
  State_psi_1d_SG_D_22_9ed94 : Inport  Port=6
  State_psi_d_SG_D_22_2f3ed : Inport  Port=7
  State_psi_fd_SG_D_22_d61c9 : Inport  Port=8
  Add_47e65 : Sum
  Add_5302b : Sum
  Add_7b312 : Sum
  Add_ac404 : Sum
  Add_e5157 : Sum
  Add_e840c : Sum
  Constant_-1_3e949 : Constant  Value=-1
  Constant_-1_7eaa8 : Constant  Value=-1
  Constant_-1_8f5ee : Constant  Value=-1
  Constant_-1_97a88 : Constant  Value=-1
  Constant_-1_c3af5 : Constant  Value=-1
  Constant_x_dd_87738 : Constant  Value=x_dd
  Constant_x_dd_987cc : Constant  Value=x_dd
  Constant_x_dd_e91a2 : Constant  Value=x_dd
  Constant_x_ddd_0b8f0 : Constant  Value=x_ddd
  Constant_x_ddd_2c262 : Constant  Value=x_ddd
  Constant_x_ddd_30aa0 : Constant  Value=x_ddd
  Constant_x_l_0422d : Constant  Value=x_l
  Constant_x_l_55ed8 : Constant  Value=x_l
  Constant_x_l_7dac2 : Constant  Value=x_l
  Constant_x_l_86146 : Constant  Value=x_l
  Constant_x_l_8c951 : Constant  Value=x_l
  Constant_x_l_b9baf : Constant  Value=x_l
  Constant_x_qd_97f19 : Constant  Value=x_qd
  Constant_x_qd_a1fc9 : Constant  Value=x_qd
  Constant_x_qd_a3274 : Constant  Value=x_qd
  Constant_x_qdd_71a58 : Constant  Value=x_qdd
  Constant_x_qdd_7a6a2 : Constant  Value=x_qdd
  Constant_x_qdd_bebc5 : Constant  Value=x_qdd
  Divide_02e83 : Product  Inputs=*/
  Divide_181c4 : Product  Inputs=*/
  Divide_adde5 : Product  Inputs=*/
  Divide_af1d6 : Product  Inputs=*/
  Divide_e0e20 : Product  Inputs=*/
  Divide_e1700 : Product  Inputs=*/
  Product_0f751 : Product
  Product_1571a : Product
  Product_35cfc : Product
  Product_48560 : Product
  Product_496b4 : Product
  Product_6bc40 : Product
  Product_88d29 : Product
  Product_9e9d2 : Product
  Product_9ecd4 : Product
  Product_d4864 : Product
  Product_d644d : Product
  Subtract_22c35 : Sum  Inputs=+-
  Subtract_2c2cb : Sum  Inputs=+-
  Subtract_53c24 : Sum  Inputs=+-
  Subtract_67b86 : Sum  Inputs=+-
  Subtract_7043c : Sum  Inputs=+-
  Subtract_a7308 : Sum  Inputs=+-
  Subtract_ab449 : Sum  Inputs=+-
  Blockout_T_e_SG_D_22_9d77c : Outport
  wires:
  State_psi_1d_SG_D_22_9ed94/1 -> Product_d644d/2
  Constant_-1_97a88/1 -> Product_496b4/1
  Subtract_a7308/1 -> Product_9e9d2/2
  Constant_x_ddd_0b8f0/1 -> Subtract_53c24/2
  Constant_x_l_55ed8/1 -> Product_496b4/2
  Constant_x_qd_a1fc9/1 -> Subtract_a7308/1
  Constant_x_l_0422d/1 -> Subtract_22c35/2
  Product_496b4/1 -> Add_47e65/1
  Constant_x_qdd_7a6a2/1 -> Subtract_a7308/2
  Add_ac404/1 -> Subtract_ab449/1
  Constant_x_l_8c951/1 -> Subtract_67b86/2
  Constant_x_qdd_71a58/1 -> Add_47e65/2
  Product_0f751/1 -> Add_7b312/1
  Constant_-1_3e949/1 -> Product_0f751/1
  Constant_x_l_b9baf/1 -> Product_0f751/2
  Product_6bc40/1 -> Add_e840c/1
  Constant_-1_8f5ee/1 -> Product_6bc40/1
  Constant_x_l_86146/1 -> Product_6bc40/2
  Product_d644d/1 -> Product_88d29/1
  Constant_-1_c3af5/1 -> Product_d644d/1
  Subtract_53c24/1 -> Product_88d29/2
  Constant_x_dd_87738/1 -> Subtract_53c24/1
  State_psi_gq_SG_D_22_ecb3d/1 -> Product_9ecd4/1
  Divide_181c4/1 -> Add_e5157/2
  Add_47e65/1 -> Product_9ecd4/2
  Constant_x_qd_97f19/1 -> Add_7b312/2
  Product_9e9d2/1 -> Divide_adde5/1
  Product_9ecd4/1 -> Divide_e0e20/1
  State_psi_kq_SG_D_22_80cd8/1 -> Product_9e9d2/1
  Divide_02e83/1 -> Add_ac404/1
  Constant_x_qd_a3274/1 -> Add_e840c/2
  Subtract_67b86/1 -> Divide_02e83/2
  Constant_x_dd_987cc/1 -> Subtract_67b86/1
  Constant_x_qdd_bebc5/1 -> Divide_af1d6/2
  Subtract_22c35/1 -> Product_1571a/2
  Constant_x_ddd_30aa0/1 -> Subtract_22c35/1
  Add_7b312/1 -> Divide_e0e20/2
  Add_e840c/1 -> Divide_adde5/2
  Add_e5157/1 -> Blockout_T_e_SG_D_22_9d77c/1
  Product_88d29/1 -> Divide_02e83/1
  Product_1571a/1 -> Divide_e1700/1
  State_psi_fd_SG_D_22_d61c9/1 -> Product_1571a/1
  Subtract_7043c/1 -> Divide_e1700/2
  Constant_x_dd_e91a2/1 -> Subtract_7043c/1
  Divide_e0e20/1 -> Subtract_2c2cb/1
  Constant_x_l_7dac2/1 -> Subtract_7043c/2
  Divide_adde5/1 -> Subtract_2c2cb/2
  Product_35cfc/1 -> Divide_181c4/1
  State_psi_q_SG_D_22_21d92/1 -> Product_35cfc/1
  State_psi_d_SG_D_22_2f3ed/1 -> Add_ac404/2
  Constant_-1_7eaa8/1 -> Product_48560/1
  Product_48560/1 -> Product_d4864/1
  State_psi_d_SG_D_22_b0899/1 -> Product_48560/2
  State_psi_q_SG_D_22_f98a6/1 -> Add_5302b/2
  Subtract_2c2cb/1 -> Add_5302b/1
  Divide_af1d6/1 -> Add_e5157/1
  Product_d4864/1 -> Divide_af1d6/1
  Divide_e1700/1 -> Subtract_ab449/2
  Add_5302b/1 -> Product_d4864/2
  Subtract_ab449/1 -> Product_35cfc/2
  Constant_x_ddd_2c262/1 -> Divide_181c4/2

== system IEEE30_case/SG_D_22/d_E_fd_SG_D_22_block ==
  note: d_E_fd_SG_D_22 in IEEE30_case
      | $\frac{V_{f,\mathrm{SG},D,22}-E_{\mathrm{fd},\mathrm{SG},D,22}\,K_{E}}{T_{E}}$
      | Automatically generated on 2025-11-01 18:36:29 .
  State_E_fd_SG_D_22_b7fa0 : Inport
  State_V_f_SG_D_22_c66fa : Inport  Port=2
  Add_0014f : Sum
  Constant_-1_7ae50 : Constant  Value=-1
  Constant_K_E_36d69 : Constant  Value=K_E
  Constant_T_E_84d6f : Constant  Value=T_E
  Divide_9c9c4 : Product  Inputs=*/
  Product_2266f : Product
  Product_2289b : Product
  Blockout_d_E_fd_SG_D_22_040cd : Outport
  wires:
  State_V_f_SG_D_22_c66fa/1 -> Add_0014f/2
  State_E_fd_SG_D_22_b7fa0/1 -> Product_2266f/2
  Constant_-1_7ae50/1 -> Product_2266f/1
  Constant_T_E_84d6f/1 -> Divide_9c9c4/2
  Product_2266f/1 -> Product_2289b/1
  Constant_K_E_36d69/1 -> Product_2289b/2
  Add_0014f/1 -> Divide_9c9c4/1
  Product_2289b/1 -> Add_0014f/1
  Divide_9c9c4/1 -> Blockout_d_E_fd_SG_D_22_040cd/1

== system IEEE30_case/SG_D_22/d_Px_1_SG_D_22_block ==
  note: d_Px_1_SG_D_22 in IEEE30_case
      | $\frac{w_{\mathrm{SG},D,22}-2\,\pi \,f_{0}}{T_{w}}-\frac{\mathrm{Px}_{1,\mathrm{SG},D,22}}{T_{w}}$
      | Automatically generated on 2025-11-01 18:36:30 .
  State_Px_1_SG_D_22_97642 : Inport
  State_w_SG_D_22_b06b5 : Inport  Port=2
  Add_1f38f : Sum
  Add_4bcee : Sum
  Constant_-1_a0bff : Constant  Value=-1
  Constant_-2.0_5d154 : Constant  Value=-2.0
  Constant_T_w_605e1 : Constant  Value=T_w
  Constant_T_w_c6433 : Constant  Value=T_w
  Constant_f0_ff22d : Constant  Value=f0
  Constant_pi_9163d : Constant  Value=pi
  Divide_3e1c8 : Product  Inputs=*/
  Divide_8b428 : Product  Inputs=*/
  Product_1f09a : Product
  Product_70952 : Product
  Product_88b24 : Product
  Blockout_d_Px_1_SG_D_22_5a954 : Outport
  wires:
  Constant_-2.0_5d154/1 -> Product_1f09a/1
  Product_1f09a/1 -> Product_70952/1
  Constant_pi_9163d/1 -> Product_1f09a/2
  Constant_f0_ff22d/1 -> Product_70952/2
  Constant_-1_a0bff/1 -> Product_88b24/1
  Product_70952/1 -> Add_4bcee/1
  State_Px_1_SG_D_22_97642/1 -> Product_88b24/2
  State_w_SG_D_22_b06b5/1 -> Add_4bcee/2
  Product_88b24/1 -> Divide_3e1c8/1
  Constant_T_w_c6433/1 -> Divide_3e1c8/2
  Add_4bcee/1 -> Divide_8b428/1
  Constant_T_w_605e1/1 -> Divide_8b428/2
  Divide_3e1c8/1 -> Add_1f38f/1
  Divide_8b428/1 -> Add_1f38f/2
  Add_1f38f/1 -> Blockout_d_Px_1_SG_D_22_5a954/1

== system IEEE30_case/SG_D_22/d_Px_2_SG_D_22_block ==
  note: d_Px_2_SG_D_22 in IEEE30_case
      | $\frac{\mathrm{Px}_{1,\mathrm{SG},D,22}-T_{2}\,\left(\frac{\mathrm{Px}_{1,\mathrm{SG},D,22}}{T_{w}}-\frac{w_{\mathrm{SG},D,22}-2\,\pi \,f_{0}}{T_{w}}\right)}{T_{1}}-\frac{\mathrm{Px}_{2,\mathrm{SG},D,22}}{T_{1}}$
      | Automatically generated on 2025-11-01 18:36:31 .
  State_Px_2_SG_D_22_a7e01 : Inport
  State_Px_1_SG_D_22_e638c : Inport  Port=2
  State_Px_1_SG_D_22_dd336 : Inport  Port=3
  State_w_SG_D_22_79a8a : Inport  Port=4
  Add_526c5 : Sum
  Add_557a7 : Sum
  Add_aaa2b : Sum
  Add_c1bd8 : Sum
  Constant_-1_5b917 : Constant  Value=-1
  Constant_-1_b301e : Constant  Value=-1
  Constant_-2.0_1ebc0 : Constant  Value=-2.0
  Constant_T_1_473e2 : Constant  Value=T_1
  Constant_T_1_b46e7 : Constant  Value=T_1
  Constant_T_2_14f5c : Constant  Value=T_2
  Constant_T_w_6576c : Constant  Value=T_w
  Constant_T_w_d9e3b : Constant  Value=T_w
  Constant_f0_ed816 : Constant  Value=f0
  Constant_pi_4ae69 : Constant  Value=pi
  Divide_2646c : Product  Inputs=*/
  Divide_28e28 : Product  Inputs=*/
  Divide_54547 : Product  Inputs=*/
  Divide_615ad : Product  Inputs=*/
  Product_1e6e7 : Product
  Product_647e2 : Product
  Product_69fc0 : Product
  Product_c24d1 : Product
  Product_d053f : Product
  Blockout_d_Px_2_SG_D_22_87151 : Outport
  wires:
  Constant_-2.0_1ebc0/1 -> Product_69fc0/1
  Add_aaa2b/1 -> Blockout_d_Px_2_SG_D_22_87151/1
  Constant_T_1_b46e7/1 -> Divide_28e28/2
  Product_1e6e7/1 -> Add_526c5/1
  Constant_pi_4ae69/1 -> Product_69fc0/2
  Product_69fc0/1 -> Product_1e6e7/1
  State_Px_1_SG_D_22_e638c/1 -> Add_557a7/1
  State_Px_1_SG_D_22_dd336/1 -> Product_c24d1/2
  Constant_f0_ed816/1 -> Product_1e6e7/2
  Constant_-1_b301e/1 -> Product_c24d1/1
  Divide_28e28/1 -> Add_aaa2b/1
  State_w_SG_D_22_79a8a/1 -> Add_526c5/2
  Product_c24d1/1 -> Divide_615ad/1
  Divide_54547/1 -> Add_aaa2b/2
  Constant_T_w_6576c/1 -> Divide_615ad/2
  State_Px_2_SG_D_22_a7e01/1 -> Product_d053f/2
  Add_526c5/1 -> Divide_2646c/1
  Constant_T_w_d9e3b/1 -> Divide_2646c/2
  Divide_615ad/1 -> Add_c1bd8/1
  Divide_2646c/1 -> Add_c1bd8/2
  Constant_T_2_14f5c/1 -> Product_647e2/1
  Add_c1bd8/1 -> Product_647e2/2
  Constant_-1_5b917/1 -> Product_d053f/1
  Product_647e2/1 -> Add_557a7/2
  Product_d053f/1 -> Divide_28e28/1
  Add_557a7/1 -> Divide_54547/1
  Constant_T_1_473e2/1 -> Divide_54547/2

== system IEEE30_case/SG_D_22/d_Px_3_SG_D_22_block ==
  note: d_Px_3_SG_D_22 in IEEE30_case
      | $\frac{\mathrm{Px}_{2,\mathrm{SG},D,22}+T_{4}\,\left(\frac{\mathrm{Px}_{1,\mathrm{SG},D,22}-T_{2}\,\left(\frac{\mathrm{Px}_{1,\mathrm{SG},D,22}}{T_{w}}-\frac{w_{\mathrm{SG},D,22}-2\,\pi \,f_{0}}{T_{w}}\right)}{T_{1}}-\frac{\mathrm{Px}_{2,\mathrm{SG},D,22}}{T_{1}}\right)}{T_{3}}-\frac{\mathrm{Px}_{3,\mathrm{SG},D,22}}{T_{3}}$
      | Automatically generated on 2025-11-01 18:36:34 .
  State_Px_3_SG_D_22_2d550 : Inport
  State_Px_2_SG_D_22_afba3 : Inport  Port=2
  State_Px_2_SG_D_22_1a197 : Inport  Port=3
  State_Px_1_SG_D_22_68613 : Inport  Port=4
  State_Px_1_SG_D_22_83b83 : Inport  Port=5
  State_w_SG_D_22_b3bb6 : Inport  Port=6
  Add_054a1 : Sum
  Add_4d25f : Sum
  Add_a91b3 : Sum
  Add_be677 : Sum
  Add_db431 : Sum
  Add_df3aa : Sum
  Constant_-1_17a62 : Constant  Value=-1
  Constant_-1_30190 : Constant  Value=-1
  Constant_-1_82c86 : Constant  Value=-1
  Constant_-2.0_006be : Constant  Value=-2.0
  Constant_T_1_14624 : Constant  Value=T_1
  Constant_T_1_ec9e7 : Constant  Value=T_1
  Constant_T_2_85579 : Constant  Value=T_2
  Constant_T_3_25078 : Constant  Value=T_3
  Constant_T_3_d5833 : Constant  Value=T_3
  Constant_T_4_2c8c2 : Constant  Value=T_4
  Constant_T_w_62dd5 : Constant  Value=T_w
  Constant_T_w_cd6b0 : Constant  Value=T_w
  Constant_f0_4483c : Constant  Value=f0
  Constant_pi_184c4 : Constant  Value=pi
  Divide_3f71c : Product  Inputs=*/
  Divide_55f57 : Product  Inputs=*/
  Divide_59edc : Product  Inputs=*/
  Divide_b0bbf : Product  Inputs=*/
  Divide_d3ed5 : Product  Inputs=*/
  Divide_fc2b1 : Product  Inputs=*/
  Product_1dc15 : Product
  Product_48385 : Product
  Product_8a7ef : Product
  Product_a27ab : Product
  Product_d8671 : Product
  Product_dd10e : Product
  Product_eee26 : Product
  Blockout_d_Px_3_SG_D_22_a3854 : Outport
  wires:
  Constant_-2.0_006be/1 -> Product_48385/1
  Constant_pi_184c4/1 -> Product_48385/2
  Product_d8671/1 -> Add_be677/1
  Product_48385/1 -> Product_d8671/1
  State_Px_1_SG_D_22_83b83/1 -> Product_dd10e/2
  Constant_f0_4483c/1 -> Product_d8671/2
  Constant_-1_30190/1 -> Product_dd10e/1
  Divide_fc2b1/1 -> Add_db431/2
  State_w_SG_D_22_b3bb6/1 -> Add_be677/2
  Product_dd10e/1 -> Divide_d3ed5/1
  Constant_T_w_62dd5/1 -> Divide_d3ed5/2
  Add_be677/1 -> Divide_fc2b1/1
  Constant_T_w_cd6b0/1 -> Divide_fc2b1/2
  Constant_T_1_ec9e7/1 -> Divide_b0bbf/2
  Divide_d3ed5/1 -> Add_db431/1
  Divide_3f71c/1 -> Add_054a1/2
  Constant_T_3_d5833/1 -> Divide_55f57/2
  Constant_T_2_85579/1 -> Product_a27ab/1
  Add_db431/1 -> Product_a27ab/2
  Constant_T_1_14624/1 -> Divide_59edc/2
  Constant_-1_82c86/1 -> Product_8a7ef/1
  Product_8a7ef/1 -> Divide_59edc/1
  State_Px_2_SG_D_22_1a197/1 -> Product_8a7ef/2
  State_Px_1_SG_D_22_68613/1 -> Add_a91b3/1
  Product_a27ab/1 -> Add_a91b3/2
  Add_054a1/1 -> Blockout_d_Px_3_SG_D_22_a3854/1
  Add_a91b3/1 -> Divide_b0bbf/1
  Divide_59edc/1 -> Add_4d25f/1
  Divide_b0bbf/1 -> Add_4d25f/2
  Product_1dc15/1 -> Add_df3aa/2
  Constant_T_4_2c8c2/1 -> Product_1dc15/1
  Add_4d25f/1 -> Product_1dc15/2
  Constant_T_3_25078/1 -> Divide_3f71c/2
  Constant_-1_17a62/1 -> Product_eee26/1
  State_Px_3_SG_D_22_2d550/1 -> Product_eee26/2
  Divide_55f57/1 -> Add_054a1/1
  Add_df3aa/1 -> Divide_3f71c/1
  State_Px_2_SG_D_22_afba3/1 -> Add_df3aa/1
  Product_eee26/1 -> Divide_55f57/1

== system IEEE30_case/SG_D_22/d_R_f_SG_D_22_block ==
  note: d_R_f_SG_D_22 in IEEE30_case
      | $-\frac{R_{f,\mathrm{SG},D,22}-\frac{E_{\mathrm{fd},\mathrm{SG},D,22}\,K_{F}}{T_{F}}}{T_{F}}$
      | Automatically generated on 2025-11-01 18:36:28 .
  State_E_fd_SG_D_22_1081a : Inport
  State_R_f_SG_D_22_53fbc : Inport  Port=2
  Constant_K_F_79e3a : Constant  Value=K_F
  Constant_T_F_9bc42 : Constant  Value=T_F
  Constant_T_F_d4c78 : Constant  Value=T_F
  Divide_4f02a : Product  Inputs=*/
  Divide_776b1 : Product  Inputs=*/
  Product_3ab5f : Product
  Subtract_ab03f : Sum  Inputs=+-
  Blockout_d_R_f_SG_D_22_62abf : Outport
  wires:
  State_E_fd_SG_D_22_1081a/1 -> Product_3ab5f/1
  Divide_776b1/1 -> Subtract_ab03f/1
  Product_3ab5f/1 -> Divide_776b1/1
  Constant_K_F_79e3a/1 -> Product_3ab5f/2
  Constant_T_F_9bc42/1 -> Divide_4f02a/2
  Constant_T_F_d4c78/1 -> Divide_776b1/2
  State_R_f_SG_D_22_53fbc/1 -> Subtract_ab03f/2
  Subtract_ab03f/1 -> Divide_4f02a/1
  Divide_4f02a/1 -> Blockout_d_R_f_SG_D_22_62abf/1

== system IEEE30_case/SG_D_22/d_T_m_SG_D_22_block ==
  note: d_T_m_SG_D_22 in IEEE30_case
      | $-\frac{T_{m,\mathrm{SG},D,22}-T_{0}+\frac{\mathrm{SpeedPara}\,\left(w_{\mathrm{SG},D,22}-w_{\mathrm{ref}}\right)}{2\,f_{0}\,\pi }}{T_{\mathrm{speed}}}$
      | Automatically generated on 2025-11-01 18:36:18 .
  State_w_SG_D_22_92dc5 : Inport
  State_T_m_SG_D_22_f2698 : Inport  Port=2
  Add_19cd1 : Sum
  Add_5ec90 : Sum
  Constant_-1_e85cf : Constant  Value=-1
  Constant_2.0_237f9 : Constant  Value=2.0
  Constant_SpeedPara_ff7a3 : Constant  Value=SpeedPara
  Constant_T_0_66a5b : Constant  Value=T_0
  Constant_T_speed_15efa : Constant  Value=T_speed
  Constant_f0_4ef57 : Constant  Value=f0
  Constant_pi_1cacf : Constant  Value=pi
  Constant_w_ref_84a81 : Constant  Value=w_ref
  Divide_83c63 : Product  Inputs=*/
  Divide_e8511 : Product  Inputs=*/
  Product_2f2a2 : Product
  Product_921ff : Product
  Product_bcb6b : Product
  Product_c015b : Product
  Subtract_e5f61 : Sum  Inputs=+-
  Blockout_d_T_m_SG_D_22_e6732 : Outport
  wires:
  Constant_SpeedPara_ff7a3/1 -> Product_921ff/1
  Constant_-1_e85cf/1 -> Product_2f2a2/1
  State_w_SG_D_22_92dc5/1 -> Product_2f2a2/2
  Constant_2.0_237f9/1 -> Product_c015b/1
  Product_2f2a2/1 -> Add_19cd1/1
  Constant_w_ref_84a81/1 -> Add_19cd1/2
  Add_19cd1/1 -> Product_921ff/2
  Constant_pi_1cacf/1 -> Product_c015b/2
  Product_c015b/1 -> Product_bcb6b/1
  Constant_f0_4ef57/1 -> Product_bcb6b/2
  Product_921ff/1 -> Divide_83c63/1
  Product_bcb6b/1 -> Divide_83c63/2
  Divide_83c63/1 -> Add_5ec90/1
  Constant_T_0_66a5b/1 -> Add_5ec90/2
  Constant_T_speed_15efa/1 -> Divide_e8511/2
  Add_5ec90/1 -> Subtract_e5f61/1
  State_T_m_SG_D_22_f2698/1 -> Subtract_e5f61/2
  Subtract_e5f61/1 -> Divide_e8511/1
  Divide_e8511/1 -> Blockout_d_T_m_SG_D_22_e6732/1
